simulink model "Etape2_simulink"  (R2022a)
settings: Solver=VariableStepAuto  StartTime=0.0  StopTime=10.0  RelTol=1e-3
settings Model: Creator=mra4306  LastModifiedBy=mra4306

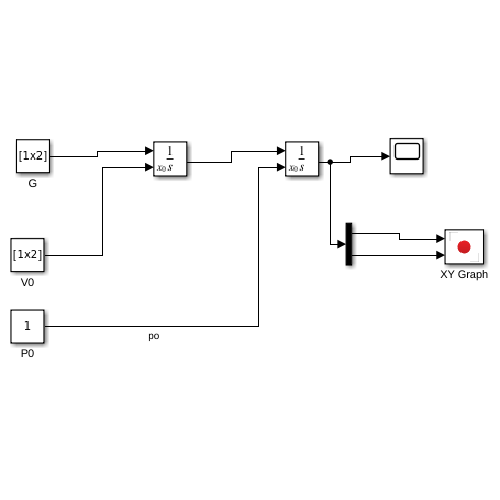
[thumbnail: Simulink's stored preview of the top-level diagram]
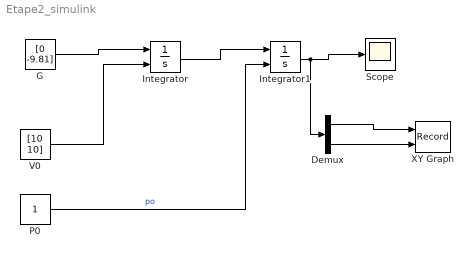
== system Etape2_simulink ==
  Demux : Demux  Outputs=2
  G : Constant  Value=[0 -9.81]
  Integrator : Integrator  InitialConditionSource=external
  Integrator1 : Integrator  InitialConditionSource=external
  P0 : Constant
  Scope : Scope
  V0 : Constant  Value=[10 10]
  XY Graph : Record  FileSettingsInternal="{\"entries\":[{\"content\":{\"excelSettings\":{\"content\":{},\"type\":\"Streamout.ExcelSettings\"}},\"type\":\"Streamout.FileSettingStorage\",\"uuid\":\"be63c21b-ac35-4d8d-9ac4-3da4b26d76fc\"}],\"packageUris\":[\"http://schema.mathworks.com/mf0/streamout_blocks/R2020a\"],\"version\":\"1.0\"}"  Layout=[1 1]  SignalsInternal="{\"entries\":[{\"content\":{\"signals\":[{\"content\":{\"blockPath\":[\"untitled/XY Graph\"],\"channel\":[],\"dimensions\":[1],\"domain\":\"untitled/XY Graph\",\"lineColor\":\"#a2142f\",\"plots\":[1],\"port\":1,\"sid\":[\"\"],\"signalID\":36,\"signalName\":\"Demux:1\"},\"type\":\"RecordBlkView.Signal\",\"uuid\":\"cdddf307-cf90-47f2-94ee-9896b94fa634\"},{\"content\":{\"blockPath\":[\"untitled/XY Graph\"],\"channel\":[],\"dimensions\":[1],\"domain\":\"untitled/XY Graph\",\"lineColor\":\"#139fff\",\"plots\":[1],\"port\":2,\"sid\":[\"\"],\"signalID\":40,\"signalName\":\"Demux:2\"},\"type\":\"RecordBlkView.Signal\",\"uuid\":\"c54cea77-9453-405f-a613-bb1f907d34af\"}]},\"type\":\"RecordBlkView.InputSignals\",\"uuid\":\"2103494a-b583-4bad-b24f-8fc02a866bde\"}],\"packageUris\":[\"http://schema.mathworks.com/mf0/streamout_blocks/R2020a\"],\"version\":\"1.0\"}"  VisualizationBindings="{\"xyplotplugin\":{\"info\":[{\"series\":[{\"bindingParametersList\":[{\"parameter\":\"X-Axis\",\"signalID\":36,\"signalName\":\"Demux:1\"},{\"parameter\":\"Y-Axis\",\"signalID\":40,\"signalName\":\"Demux:2\"}],\"seriesID\":24348}],\"subplotID\":1}]}}"  CompatibilityTag=XY
  wires:
  G/1 -> Integrator/1
  V0/1 -> Integrator/2
  Integrator/1 -> Integrator1/1
  P0/1 -> Integrator1/2  "po"
  Integrator1/1 -> Demux/1, Scope/1
  Demux/2 -> XY Graph/2
  Demux/1 -> XY Graph/1
